simulink model "Compensator_Design_for_the_PLL"  (R2021a)
settings: Solver=ode23tb  StartTime=0.0  StopTime=2  FixedStep=50e-6  MaxStep=1e-3  RelTol=1e-4  EnableMultiTasking=on
PreLoadFcn:
  | Ts=0;
libraries: powerlib_meascontrol x2, spsThreePhaseProgrammableGeneratorLib x2, spsabctodq0Lib x2
Description:
  | Copyright 2008-2015 The MathWorks, Inc.
settings Model: Creator=MathWorks  LastModifiedBy=aks
settings SolverCC: AlgebraicLoopSolver=TrustRegion
settings DataIOCC: LimitDataPoints=on  SaveFormat=Array  SignalLoggingSaveFormat=ModelDataLogs  ReturnWorkspaceOutputs=off
settings OptimizationCC: ExpressionDepthLimit=2147483647  LifeSpan=inf
settings DebuggingCC: ReadBeforeWriteMsg=DisableAll  WriteAfterWriteMsg=DisableAll  WriteAfterReadMsg=DisableAll  UnderspecifiedInitializationDetection=Classic  MergeDetectMultiDrivingBlocksExec=none  SolverPrmCheckMsg=warning  FcnCallInpInsideContextMsg=warning  AllowSymbolicDim=off  StateNameClashWarn=warning  SFUnexpectedBacktrackingDiag=warning  SFNoUnconditionalDefaultTransitionDiag=warning  SFExecutionAtInitializationDiag=none  SFMachineParentedDataDiag=warning  ArithmeticOperatorsInVariantConditions=warning
settings HardwareCC: ProdBitPerPointer=32  ProdBitPerSizeT=32  ProdBitPerPtrDiffT=32  ProdLargestAtomicFloat=None  ProdIntDivRoundTo=Undefined  ProdEndianess=Unspecified  ProdWordSize=32  ProdHWDeviceType=32-bit Generic
settings ModelReferenceCC: PropagateSignalLabelsOutOfModel=off
settings SFSimCC: SimUseLocalCustomCode=off  CustomCodeUndefinedFunction=UseInterfaceOnly
settings RTWCC: RTWUseLocalCustomCode=off
settings CodeAppCC: StateflowObjectComments=on
settings GRTTargetCC: TargetLangStandard=C89/C90 (ANSI)
settings ConfigComp: CovMetricSettings=dw  CovSaveCumulativeToWorkspaceVar=on  CovSaveSingleToWorkspaceVar=on  CovExternalEMLEnable=off  CovSFcnEnable=off
settings SimscapeCC: SimscapeNormalizeSystem=off

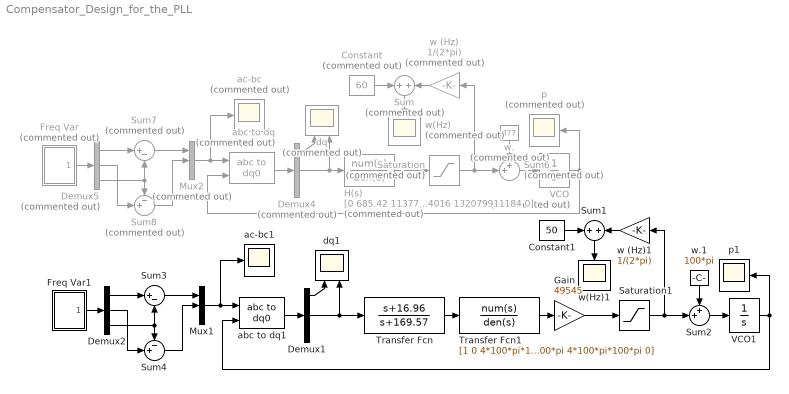
== system Compensator_Design_for_the_PLL ==
  Constant : Constant  Commented=on  Value=60
  Constant1 : Constant  Value=50
  Demux1 : Demux  Outputs=3
  Demux2 : Demux  Outputs=3
  Demux4 : Demux  Commented=on  Outputs=3
  Demux5 : Demux  Commented=on  Outputs=3
  Freq Var : Subsystem  Commented=on
  Freq Var1 : Subsystem
  Gain : Gain  Gain=49545
  H(s) : TransferFcn  Commented=on  Numerator=[0 685.42 113779.72 394394095.1 64685591295.52 2684452038764.08]  Denominator=[1 2472 2254552 898394016 132079911184 0]
  Mux1 : Mux  Inputs=3
  Mux2 : Mux  Commented=on  Inputs=3
  Saturation : Saturate  Commented=on  UpperLimit=500  LowerLimit=-500
  Saturation1 : Saturate  UpperLimit=500  LowerLimit=-500
  Sum : Sum  Commented=on  Inputs=+|+
  Sum1 : Sum  Inputs=+|+
  Sum2 : Sum  Inputs=++|
  Sum3 : Sum  Inputs=|+-
  Sum4 : Sum  Inputs=-+|
  Sum6 : Sum  Commented=on  Inputs=++|
  Sum7 : Sum  Commented=on  Inputs=|+-
  Sum8 : Sum  Commented=on  Inputs=-+|
  Transfer Fcn : TransferFcn  Numerator=[1 16.96]  Denominator=[1 169.57]
  Transfer Fcn1 : TransferFcn  Numerator=[1 0 4*100*pi*100*pi]  Denominator=[1 4*100*pi 4*100*pi*100*pi 0]
  VCO : Integrator  Commented=on  UpperSaturationLimit=2*pi  LowerSaturationLimit=0  WrapState=on  WrappedStateUpperValue=2*pi  WrappedStateLowerValue=0
  VCO1 : Integrator  UpperSaturationLimit=2*pi  LowerSaturationLimit=0  WrapState=on  WrappedStateUpperValue=2*pi  WrappedStateLowerValue=0
  abc to dq : spsabctodq0Lib/abc to dq0  Commented=on  Alignment=90 degrees behind phase A axis
  abc to dq1 : spsabctodq0Lib/abc to dq0  Alignment=90 degrees behind phase A axis
  ac-bc : Scope  Commented=on
  ac-bc1 : Scope
  dq : Scope  Commented=on  NumInputPorts=2
  dq1 : Scope  NumInputPorts=2
  p : Scope  Commented=on
  p1 : Scope
  w (Hz) : Gain  Commented=on  Gain=1/(2*pi)
  w (Hz)1 : Gain  Gain=1/(2*pi)
  w(Hz) : Scope  Commented=on
  w(Hz)1 : Scope
  w. : Constant  Commented=on  Value=377
  w.1 : Constant  Value=100*pi
  wires:
  Saturation/1 -> w (Hz)/1, Sum6/2
  H(s)/1 -> Saturation/1
  abc to dq/1 -> Demux4/1
  Sum6/1 -> VCO/1
  Demux4/2 -> dq/2, H(s)/1
  VCO/1 -> p/1, abc to dq/2
  w./1 -> Sum6/1
  Demux4/1 -> dq/1
  Demux5/1 -> Sum7/1
  Sum7/1 -> Mux2/1
  Sum8/1 -> Mux2/2
  Demux5/3 -> Sum8/1, Sum7/2
  Demux5/2 -> Sum8/2
  Freq Var/1(abc) -> Demux5/1
  Mux2/1 -> abc to dq/1, ac-bc/1
  Sum/1 -> w(Hz)/1
  w (Hz)/1 -> Sum/2
  Constant/1 -> Sum/1
  Constant1/1 -> Sum1/1
  w (Hz)1/1 -> Sum1/2
  Sum1/1 -> w(Hz)1/1
  Mux1/1 -> ac-bc1/1, abc to dq1/1
  Freq Var1/1(abc) -> Demux2/1
  Demux2/2 -> Sum4/2
  Demux2/3 -> Sum3/2, Sum4/1
  Sum4/1 -> Mux1/2
  Sum3/1 -> Mux1/1
  Demux2/1 -> Sum3/1
  Demux1/1 -> dq1/1
  w.1/1 -> Sum2/1
  VCO1/1 -> abc to dq1/2, p1/1
  Demux1/2 -> Transfer Fcn/1, dq1/2
  Sum2/1 -> VCO1/1
  abc to dq1/1 -> Demux1/1
  Gain/1 -> Saturation1/1
  Saturation1/1 -> Sum2/2, w (Hz)1/1
  Transfer Fcn1/1 -> Gain/1
  Transfer Fcn/1 -> Transfer Fcn1/1

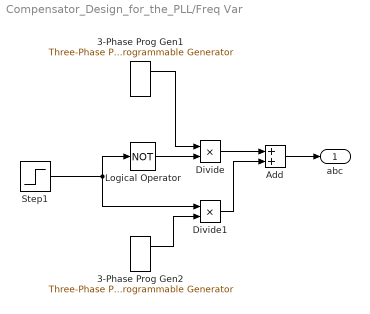
== system Compensator_Design_for_the_PLL/Freq Var ==
  3-Phase Prog Gen1 : powerlib_meascontrol/Pulse & Signal Generators/Three-Phase Programmable Generator  Par_Vps=[391 0 60]  VariationEntity=Frequency  VariationType=Step  VariationStep=3  VariationRate=10  VariationMag=0.3  VariationFreq=2  Par_Timing_Variation="[0.45  0.5  ]"  SinglePhase=off  Yampli=[0 3 3 -3]  Xtime=[0 0.45 0.5 0.55]  HarmonicGeneration=off  Par_HarmoA="[1  130  0 2]"  Par_HarmoB="[1  0  0 1]"  Par_Timing_Harmo="[0.25  0.35]"  Ts=0
      settings: SourceProductBaseCode=PS
  3-Phase Prog Gen2 : powerlib_meascontrol/Pulse & Signal Generators/Three-Phase Programmable Generator  Par_Vps=[391 0 60.3]  VariationEntity=Frequency  VariationType=Step  VariationStep=-3.3  VariationRate=10  VariationMag=0.3  VariationFreq=2  Par_Timing_Variation="[0.5  0.65]"  SinglePhase=on  Yampli=[1 0.2 1.2 1.0]  Xtime=[0 0.1 0.15 0.2]  HarmonicGeneration=off  Par_HarmoA="[1  130  0 2]"  Par_HarmoB="[1  0  0 1]"  Par_Timing_Harmo="[0.25  0.35]"  Ts=0
      settings: SourceProductBaseCode=PS
  Add : Sum
  Divide : Product  Inputs=**
  Divide1 : Product  Inputs=**
  Logical Operator : Logic  Operator=NOT  AllPortsSameDT=off  OutDataTypeStr=boolean
  Step1 : Step  Time=0.5  SampleTime=0
  abc : Outport
  wires:
  Step1/1 -> Logical Operator/1, Divide1/1
  Divide/1 -> Add/1
  Divide1/1 -> Add/2
  3-Phase Prog Gen1/1 -> Divide/1
  3-Phase Prog Gen2/1 -> Divide1/2
  Add/1 -> abc/1
  Logical Operator/1 -> Divide/2

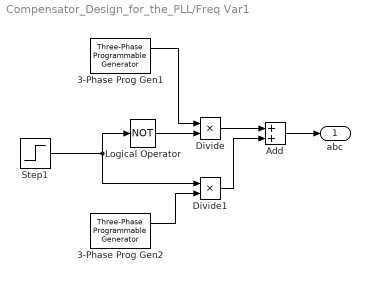
== system Compensator_Design_for_the_PLL/Freq Var1 ==
  3-Phase Prog Gen1 : spsThreePhaseProgrammableGeneratorLib/Three-Phase Programmable Generator  Par_Vps=[1 0 50]  VariationEntity=Frequency  VariationType=Step  VariationStep=5  VariationRate=10  VariationMag=0.3  VariationFreq=2  Par_Timing_Variation="[0.15  0.3  ]"  SinglePhase=off  Yampli=[0 3 3 -3]  Xtime=[0 0.45 0.5 0.55]  HarmonicGeneration=off  Par_HarmoA="[1  130  0 2]"  Par_HarmoB="[1  0  0 1]"  Par_Timing_Harmo="[0.25  0.35]"  Ts=0
      settings: SourceProductBaseCode=PS
  3-Phase Prog Gen2 : spsThreePhaseProgrammableGeneratorLib/Three-Phase Programmable Generator  Par_Vps=[1 0 50]  VariationEntity=Frequency  VariationType=Step  VariationStep=-5  VariationRate=10  VariationMag=0.3  VariationFreq=2  Par_Timing_Variation="[0.7  1.5]"  SinglePhase=on  Yampli=[1 0.2 1.2 1.0]  Xtime=[0 0.1 0.15 0.2]  HarmonicGeneration=off  Par_HarmoA="[1  130  0 2]"  Par_HarmoB="[1  0  0 1]"  Par_Timing_Harmo="[0.25  0.35]"  Ts=0
      settings: SourceProductBaseCode=PS
  Add : Sum
  Divide : Product  Inputs=**
  Divide1 : Product  Inputs=**
  Logical Operator : Logic  Operator=NOT  AllPortsSameDT=off  OutDataTypeStr=boolean
  Step1 : Step  Time=0.5  SampleTime=0
  abc : Outport
  wires:
  Logical Operator/1 -> Divide/2
  Add/1 -> abc/1
  3-Phase Prog Gen2/1 -> Divide1/2
  3-Phase Prog Gen1/1 -> Divide/1
  Divide1/1 -> Add/2
  Divide/1 -> Add/1
  Step1/1 -> Divide1/1, Logical Operator/1
